simulink model "ram2"  (R2022b)
settings: Solver=VariableStepAuto  StartTime=0.0  StopTime=inf  RelTol=1e-3
libraries: hdlsllib x1
settings Model: Creator=F1  LastModifiedBy=Namratha
settings SolverCC: AlgebraicLoopSolver=TrustRegion
settings DebuggingCC: UnconnectedInputMsg=warning  UnconnectedOutputMsg=warning  UnconnectedLineMsg=warning  SFMachineParentedDataDiag=warning
settings ModelReferenceCC: EnableRefExpFcnMdlSchedulingChecks=on

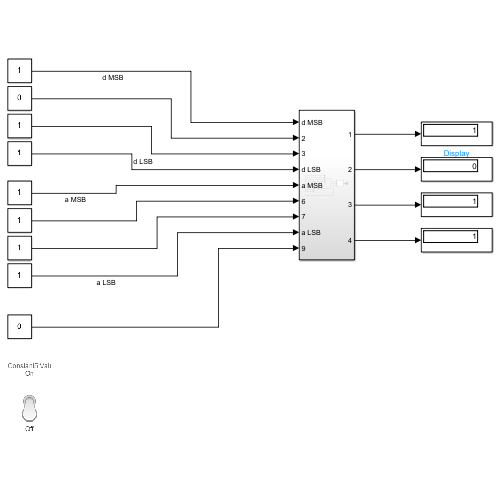
[thumbnail: Simulink's stored preview of the top-level diagram]
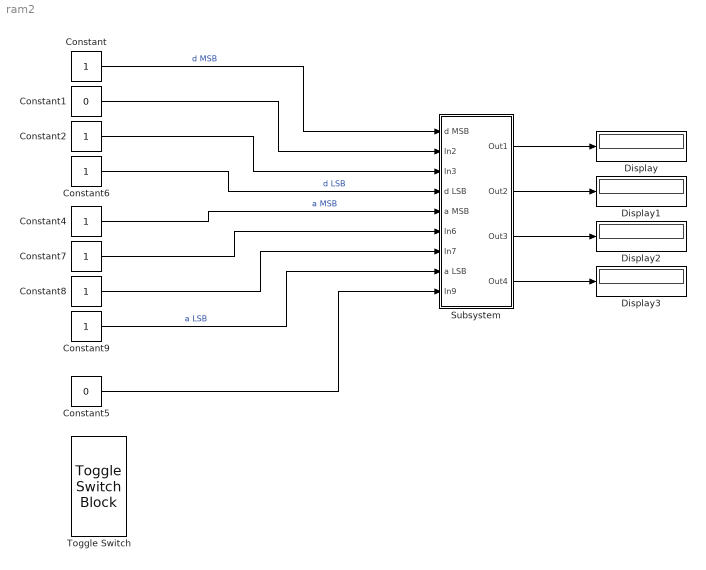
== system ram2 ==
  Constant{,2,4,6..9} (7 alike) : Constant
  Constant1 : Constant  Value=0
  Constant5 : Constant  Value=0
  Display{,1..3} (4 alike) : Display
  Subsystem : Subsystem
  Toggle Switch : ToggleSwitchBlock
      settings: Values={{'Off', 'On'}, [0 1]}
  wires:
  Constant/1 -> Subsystem/1(d MSB)  "d MSB"
  Constant1/1 -> Subsystem/2(In2)
  Constant2/1 -> Subsystem/3(In3)
  Constant6/1 -> Subsystem/4(d LSB)  "d LSB"
  Constant4/1 -> Subsystem/5(a MSB)  "a MSB"
  Constant7/1 -> Subsystem/6(In6)
  Constant8/1 -> Subsystem/7(In7)
  Constant9/1 -> Subsystem/8(a LSB)  "a LSB"
  Constant5/1 -> Subsystem/9(In9)
  Subsystem/1(Out1) -> Display/1
  Subsystem/2(Out2) -> Display1/1
  Subsystem/3(Out3) -> Display2/1
  Subsystem/4(Out4) -> Display3/1

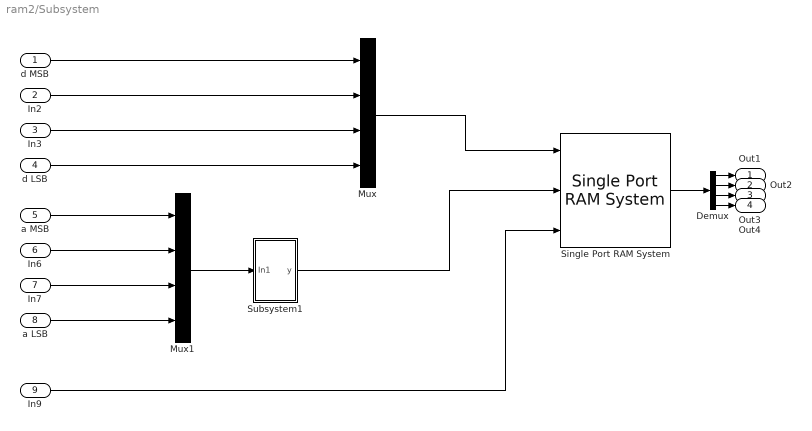
== system ram2/Subsystem ==
  d MSB : Inport
  In2 : Inport  Port=2
  In3 : Inport  Port=3
  d LSB : Inport  Port=4
  a MSB : Inport  Port=5
  In6 : Inport  Port=6
  In7 : Inport  Port=7
  a LSB : Inport  Port=8
  In9 : Inport  Port=9
  Demux : Demux
  Mux : Mux
  Mux1 : Mux
  Single Port RAM System : hdlsllib/HDL RAMs/Single Port RAM System  RAMType=Single port  WriteOutputValue=New data  RAMInitialValue=0  SimulateUsing=Code generation
  Subsystem1 : Subsystem
  Out1 : Outport
  Out2 : Outport  Port=2
  Out3 : Outport  Port=3
  Out4 : Outport  Port=4
  wires:
  a LSB/1 -> Mux1/4
  In7/1 -> Mux1/3
  In2/1 -> Mux/2
  a MSB/1 -> Mux1/1
  Subsystem1/1(y) -> Single Port RAM System/2
  d LSB/1 -> Mux/4
  Mux/1 -> Single Port RAM System/1
  In9/1 -> Single Port RAM System/3
  Mux1/1 -> Subsystem1/1(In1)
  Demux/1 -> Out1/1
  Single Port RAM System/1 -> Demux/1
  d MSB/1 -> Mux/1
  In3/1 -> Mux/3
  In6/1 -> Mux1/2
  Demux/2 -> Out2/1
  Demux/3 -> Out3/1
  Demux/4 -> Out4/1

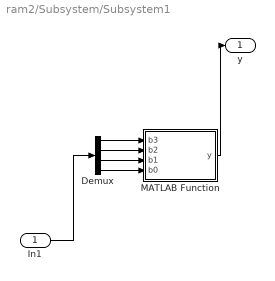
== system ram2/Subsystem/Subsystem1 ==
  In1 : Inport
  Demux : Demux
  MATLAB Function : MATLAB Function  TreatAsAtomicUnit=on
  y : Outport
  wires:
  Demux/3 -> MATLAB Function/3(b1)
  Demux/1 -> MATLAB Function/1(b3)
  Demux/2 -> MATLAB Function/2(b2)
  Demux/4 -> MATLAB Function/4(b0)
  MATLAB Function/1(y) -> y/1
  In1/1 -> Demux/1

== matlab function ram2/Subsystem/Subsystem1/MATLAB Function ==
  data: b3 input; y output; b2 input; b1 input; b0 input
function y = fcn( b3   , b2   , b1    , b0    )
y =  b3*2^3 + b2*2^2 + b1*2^1 + b0*2^0 ;
end
